simulink library "correlator_library"  (Simulink 6.2)
values from neighbouring files (symbols this model uses):
  AntBits = ceil(log2(AntNum))    [x_engine_mask.m]
  AntNum = 2    [x_engine_mask.m]
  BitGrowth = ceil(log2(AccLen))    [x_engine_mask.m]
undefined symbols (not defined in the file or in its folder): AccLen, add_latency, BitWidthIn, BitWidthOut, mult_latency
libraries: xbsIndex_r3 x745, correlator_library x7, delay_lib x5, xps_library x4
(part 1 of 6)
settings Model: LastModifiedBy=aparsons

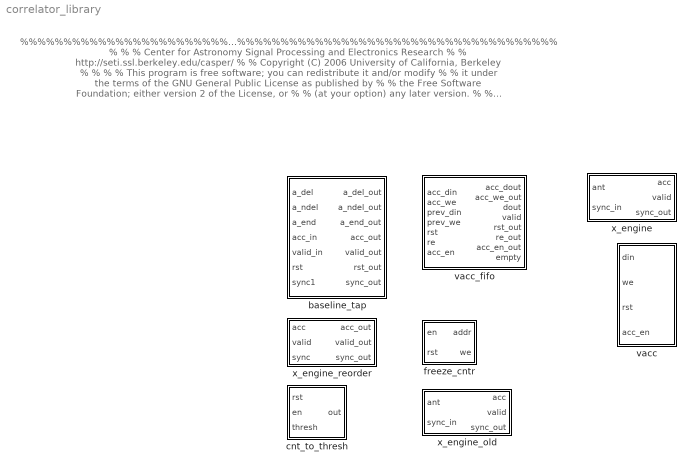
== system correlator_library ==
  note: %%%%%%%%%%%%%%%%%%%%%%%%%%%%%%%%%%%%%%%%%%%%%%%%%%%%%%%%%%%%%%%%%%%%%%%%%%%%%%%
      | %                                                                             %
      | %   Center for Astronomy Signal Processing and Electronics Research           %
      | %   http://seti.ssl.berkeley.edu/casper/                                      %
      | %   Copyright (C) 2006 University of California, Berkeley                     %
      | %                                                                             %
      | %   This program is free software; you can redistribute it and/or modify      %
      | %   it under the terms of the GNU General Public License as published by      %
      | %   the Free Software Foundation; either version 2 of the License, or         %
      | %   (at your option) any later version.                                       %
      | %                                                                             %
      | %   This program is distributed in the hope that it will be useful,           %
      | %   but WITHOUT ANY WARRANTY; without even the implied warranty of            %
      | %   MERCHANTABILITY or FITNESS FOR A PARTICULAR PURPOSE.  See the             %
      | %   GNU General Public License for more details.                              %
      | %                                                                             %
      | %   You should have received a copy of the GNU General Public License along   %
      | %   with this program; if not, write to the Free Software Foundation, Inc.,   %
      | %   51 Franklin Street, Fifth Floor, Boston, MA 02110-1301 USA.               %
      | %                                                                             %
      | %%%%%%%%%%%%%%%%%%%%%%%%%%%%%%%%%%%%%%%%%%%%%%%%%%%%%%%%%%%%%%%%%%%%%%%%%%%%%%%
  baseline_tap : Subsystem  mask(x_engine_tap){AntSep=8, use_mult_core=off, use_bram=off}
      mask prompts: AntSep "Antenna Seperation"; use_mult_core "Use Dedicated Multiplers"; use_bram "Delay in BRAM"
      mask init:
      | cursys = gcb;
      | disp(cursys);
      | multipliers = find_system(cursys, 'lookUnderMasks', 'all', 'FollowLinks','on', 'masktype', 'Xilinx Multiplier');
      | if ~strcmp(get_param(multipliers{1}, 'use_embedded'), use_mult_core),
      |     for i=1:length(multipliers),
      |         set_param(multipliers{i}, 'use_embedded', use_mult_core);
      |     end
      | end
      | if use_bram,
      |     delay_type = 'delay_bram';
      | else,
      |     delay_type = 'delay_slr';
      | end
      | if ~strcmp(get_param([cursys,'/delay'], 'BlockChoice'), delay_type),
      |     set_param([cursys,'/delay'], 'BlockChoice', delay_type)
      | end
  cnt_to_thresh : Subsystem  mask{tot_bits=0}
      mask prompts: tot_bits "Counter Bit Width"
  freeze_cntr : Subsystem  mask{CounterBits=11}
      mask prompts: CounterBits "Counter Length (2^?)"
  vacc : Subsystem  mask{vlen=8, n_bits=32, bin_pt=0, add_latency=2, arith_type=Unsigned, BitWidthIn=3, BinPtIn=0, streams=2}
      mask prompts: vlen "Vector Length"; n_bits "Output Sample Bit Width"; bin_pt "Output Binary Point"; add_latency "Add Latency"; arith_type "Arithmetic Type"; BitWidthIn "Input Bit Width"; BinPtIn "Input Binary Point"; streams "Number of Parallel Streams"
      mask init:
      | cursys = gcb;
      | disp(cursys);
      | 
      | core = [cursys,'/acc_core'];
      | if ~strcmp(get_param(core, 'arith_type'), arith_type),
      |     set_param(core, 'arith_type', arith_type);
      | end
      mask StyleString: edit,edit,edit,edit,popup(Unsigned|Signed  (2's comp)),edit,edit,edit
  vacc_fifo : Subsystem  mask(vacc_fifo){vlen=0, n_bits=0, bin_pt=0, add_latency=0, arith_type=Unsigned, BitWidthIn=0, BinPtIn=0, streams=2, stream=1}
      mask prompts: vlen "Vector Length"; n_bits "Output Sample Bit Width"; bin_pt "Output Binary Point"; add_latency "Add Latency"; arith_type "Arithmetic Type"; BitWidthIn "Input Bit Width"; BinPtIn "Input Binary Point"; streams "Number of Parallel Streams"; stream "Stream Number"
      mask init:
      | cursys = gcb;
      | disp(cursys);
      | 
      | fifo_bits = ceil(log2(max(vlen, 16)));
      | if fifo_bits >= 10,
      |     fifo_str = [num2str(2^(fifo_bits-10)), 'K'];
      | else,
      |     fifo_str = num2str(2^fifo_bits);
      | end
      | fifos = find_system(cursys, 'lookUnderMasks', 'all', 'FollowLinks','on', 'SearchDepth', 1, ...
      |     'masktype', 'Xilinx Synchronous FIFO');
      | if ~strcmp(get_param(fifos{1}, 'depth'), fifo_str),
      |     for i=1:length(fifos),
      |         set_param(fifos{i}, 'depth', fifo_str);
      |     end
      | end
      | arith_blks = {'constant', 'acc', 'reint'};
      | for i=1:length(arith_blks),
      |     name = [cursys,'/',arith_blks{i}];
      |     if ~strcmp(get_param(name, 'arith_type'), arith_type),
      |         set_param(name, 'arith_type', arith_type);
      |     end
      | end
      mask StyleString: edit,edit,edit,edit,popup(Unsigned|Signed  (2's comp)),edit,edit,edit,edit
  x_engine : Subsystem  mask{AntNum=5, BitWidthIn=8, BitWidthOut=18, AccLen=32, add_latency=1, mult_latency=1, bram_latency=1, use_mult_core=on, use_bram=off}
      mask prompts: AntNum "Number of Antennas"; BitWidthIn "Bit Width of Samples In"; BitWidthOut "Bit Width of Samples Out"; AccLen "Accumulation Length"; add_latency "Add Latency"; mult_latency "Mult Latency"; bram_latency "BRAM Latency"; use_mult_core "Use Dedicated Multipliers"; use_bram "Delay in BRAM"
      mask init:
      | x_engine_mask;
  x_engine_old : Subsystem  mask{AntNum=5, BitWidthIn=18, BitWidthOut=18, AccLen=32, add_latency=2, mult_latency=3, bram_latency=2, use_mult_core=on}
      mask prompts: AntNum "Number of Antennas"; BitWidthIn "Bit Width of Samples In"; BitWidthOut "Bit Width of Samples Out"; AccLen "Accumulation Length"; add_latency "Add Latency"; mult_latency "Mult Latency"; bram_latency "BRAM Latency"; use_mult_core "Use Dedicated Multipliers"
      mask init:
      | cursys = gcb;
      | disp(cursys);
      | set_param([cursys,'/x_engine_core'], 'use_mult_core', use_mult_core);
  x_engine_reorder : Subsystem  mask{num_ants=5, acc_len=8}
      mask prompts: num_ants "Number of Antennas"; acc_len "X Engine Accumulation Length"
      mask init:
      | num_taps = floor(num_ants/2) + 1;
      | toggle_len = num_ants * acc_len * 2;
      | 
      | addr_offset = floor(num_ants/2) * num_taps - sum(1:num_taps-1) - 1;
      | if (mod(num_ants, 2) == 0)
      |     addr_offset = addr_offset - floor(num_ants/2);
      | end
      | 
      | num_elements = nchoosek(num_ants, 2) + num_ants;
      | elements_bits = floor(log2(num_elements)) + 1;
      | %num_valids = floor(num_ants/2) + num_ants;
      | %valid_len = num_valids * acc_len;

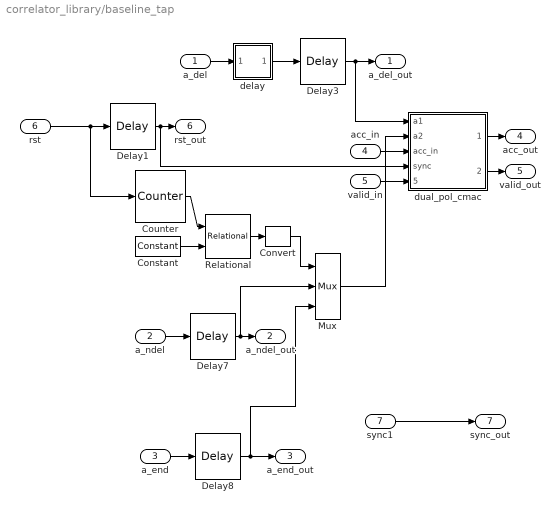
== system correlator_library/baseline_tap ==
  a_del : Inport  Port=1  LatchInput=off
  a_ndel : Inport  Port=2  LatchInput=off
  a_end : Inport  Port=3  LatchInput=off
  acc_in : Inport  Port=4  LatchInput=off
  valid_in : Inport  Port=5  LatchInput=off
  rst : Inport  Port=6  LatchInput=off
  sync1 : Inport  Port=7  LatchInput=off
  Constant : xbsIndex_r3/Constant  const=AntSep * AccLen  equ=P=C  arith_type=Unsigned  n_bits=AntBits + BitGrowth  bin_pt=0  opselect=C  inp2=PCIN>>17  opr=+  inp1=P  carry=CIN  iostate=0  explicit_period=off  period=1  dbl_ovrd=off
  Convert : xbsIndex_r3/Convert  arith_type=Unsigned  n_bits=1  bin_pt=0  quantization=Truncate  overflow=Wrap  latency=0  explicit_period=off  period=1  dbl_ovrd=off  show_param=off  inserted_by_tool=off  pipeline=off
      settings: xl_area=[0, 0, 0, 0, 0, 0, 0]
  Counter : xbsIndex_r3/Counter  cnt_type=Count Limited  n_bits=AntBits + BitGrowth  bin_pt=0  arith_type=Unsigned  start_count=0  cnt_to=AntNum * AccLen - 1  cnt_by_val=1  operation=Up  explicit_period=off  period=1  load_pin=off  rst=on  en=off  dbl_ovrd=off  show_param=off  use_rpm=on  gen_core=off
      settings: xl_area=[0, 0, 0, 0, 0, 0, 0]
  Delay1 : xbsIndex_r3/Delay  latency=1  reg_retiming=off  explicit_period=off  period=1  en=off  accept_only_valid=off  init_zero=on  dbl_ovrd=off  show_param=off
      settings: xl_area=[0, 0, 0, 0, 0, 0, 0]
  Delay3 : xbsIndex_r3/Delay  latency=1  reg_retiming=off  explicit_period=off  period=1  en=off  accept_only_valid=off  init_zero=on  dbl_ovrd=off  show_param=off
      settings: xl_area=[0, 0, 0, 0, 0, 0, 0]
  Delay7 : xbsIndex_r3/Delay  latency=1  reg_retiming=off  explicit_period=on  period=1  en=off  accept_only_valid=off  init_zero=on  dbl_ovrd=off  show_param=off
      settings: xl_area=[0, 0, 0, 0, 0, 0, 0]
  Delay8 : xbsIndex_r3/Delay  latency=1  reg_retiming=off  explicit_period=on  period=1  en=off  accept_only_valid=off  init_zero=on  dbl_ovrd=off  show_param=off
      settings: xl_area=[0, 0, 0, 0, 0, 0, 0]
  Mux : xbsIndex_r3/Mux  inputs=2  precision=Full  arith_type="Signed  (2's comp)"  n_bits=8  bin_pt=2  quantization=Truncate  overflow=Wrap  latency=0  explicit_period=off  period=1  en=off  dbl_ovrd=off  show_param=off  mux_type=off  use_rpm=off  gen_core=off
      settings: xl_area=[0, 0, 0, 0, 0, 0, 0]
  Relational : xbsIndex_r3/Relational  mode=a<b  latency=1  explicit_period=off  period=1  en=off  dbl_ovrd=off  show_param=off
      settings: xl_area=[0, 0, 0, 0, 0, 0, 0]
  delay : Subsystem  BlockChoice=delay_slr
      link override delay_bram: DelayLen=AccLen  bram_latency=bram_latency
      link override delay_bram/Constant2: equ=P=C
      link override delay_slr: DelayLen=AccLen
      settings: AttributesFormatString=%<BlockChoice>  TemplateBlock=delay_lib/delay  MemberBlocks=delay_bram,delay_slr
  dual_pol_cmac : Subsystem
  a_del_out : Outport
  a_ndel_out : Outport  Port=2
  a_end_out : Outport  Port=3
  acc_out : Outport  Port=4
  valid_out : Outport  Port=5
  rst_out : Outport  Port=6
  sync_out : Outport  Port=7
  wires:
  delay/1(Out1) -> Delay3/1
  Mux/1 -> dual_pol_cmac/2(a2)
  Counter/1 -> Relational/1
  Constant/1 -> Relational/2
  Relational/1 -> Convert/1
  Convert/1 -> Mux/1
  rst/1 -> Delay1/1, Counter/1
  a_del/1 -> delay/1(In1)
  dual_pol_cmac/1(acc_out) -> acc_out/1
  acc_in/1 -> dual_pol_cmac/3(acc_in)
  dual_pol_cmac/2(valid_out) -> valid_out/1
  valid_in/1 -> dual_pol_cmac/5(valid_in)
  a_ndel/1 -> Delay7/1
  a_end/1 -> Delay8/1
  Delay3/1 -> a_del_out/1, dual_pol_cmac/1(a1)
  Delay7/1 -> a_ndel_out/1, Mux/2
  Delay8/1 -> a_end_out/1, Mux/3
  Delay1/1 -> rst_out/1, dual_pol_cmac/4(sync)
  sync1/1 -> sync_out/1

== system correlator_library/cnt_to_thresh ==
  rst : Inport  Port=1  LatchInput=off
  en : Inport  Port=2  LatchInput=off
  thresh : Inport  Port=3  LatchInput=off
  Inverter : xbsIndex_r3/Inverter  latency=0  explicit_period=off  period=1  en=off  dbl_ovrd=off  show_param=off
      settings: xl_area=[0, 0, 0, 0, 0, 0, 0]
  Logical : xbsIndex_r3/Logical  logical_function=AND  inputs=3  precision=Full  arith_type=Unsigned  n_bits=8  bin_pt=2  align_bp=on  latency=0  explicit_period=off  period=1  en=off  dbl_ovrd=off  show_param=off
      settings: xl_area=[0, 0, 0, 0, 0, 0, 0]
  Logical1 : xbsIndex_r3/Logical  logical_function=OR  inputs=2  precision=Full  arith_type=Unsigned  n_bits=8  bin_pt=2  align_bp=on  latency=0  explicit_period=off  period=1  en=off  dbl_ovrd=off  show_param=off
      settings: xl_area=[0, 0, 0, 0, 0, 0, 0]
  Relational1 : xbsIndex_r3/Relational  mode=a>=b  latency=2  explicit_period=on  period=1  en=on  dbl_ovrd=off  show_param=off
      settings: xl_area=[0, 0, 0, 0, 0, 0, 0]
  accumulator_adder1 : xbsIndex_r3/AddSub  mode=Subtraction  precision=User Defined  arith_type=Unsigned  n_bits=tot_bits  bin_pt=0  quantization=Truncate  overflow=Wrap  latency=add_latency  explicit_period=on  period=1  use_carryin=off  use_carryout=off  en=off  dbl_ovrd=off  show_param=off  use_core=on  pipeline=off  use_rpm=on  gen_core=off
      settings: xl_area=[0, 0, 0, 0, 0, 0, 0]
  accumulator_address_delay : xbsIndex_r3/Delay  latency=1  reg_retiming=off  explicit_period=off  period=1  en=on  accept_only_valid=off  init_zero=on  dbl_ovrd=off  show_param=off
      settings: xl_area=[0, 0, 0, 0, 0, 0, 0]
  const_accumulator_data_reset1 : xbsIndex_r3/Constant  const=2 + 1  equ=P=C  arith_type=Unsigned  n_bits=n_bits  bin_pt=0  opselect=C  inp2=PCIN>>17  opr=+  inp1=P  carry=CIN  iostate=0  explicit_period=on  period=1  dbl_ovrd=off
  int_cnt : xbsIndex_r3/Counter  cnt_type=Free Running  n_bits=tot_bits  bin_pt=0  arith_type=Unsigned  start_count=0  cnt_to=Inf  cnt_by_val=1  operation=Up  explicit_period=off  period=1  load_pin=off  rst=on  en=on  dbl_ovrd=off  show_param=off  use_rpm=on  gen_core=off
      settings: xl_area=[0, 0, 0, 0, 0, 0, 0]
  out : Outport
  wires:
  Inverter/1 -> Logical/2
  accumulator_address_delay/1 -> Inverter/1
  Logical1/1 -> int_cnt/1
  int_cnt/1 -> Relational1/1, out/1
  accumulator_adder1/1 -> Relational1/2
  const_accumulator_data_reset1/1 -> accumulator_adder1/2
  rst/1 -> Logical1/2
  en/1 -> accumulator_address_delay/2, Logical/3, int_cnt/2, Relational1/3
  thresh/1 -> accumulator_adder1/1
  Logical/1 -> Logical1/1
  Relational1/1 -> accumulator_address_delay/1, Logical/1

== system correlator_library/freeze_cntr ==
  en : Inport  Port=1  LatchInput=off
  rst : Inport  Port=2  LatchInput=off
  Constant5 : xbsIndex_r3/Constant  const=2^CounterBits - 1  equ=P=C  arith_type=Unsigned  n_bits=CounterBits  bin_pt=0  opselect=C  inp2=PCIN>>17  opr=+  inp1=P  carry=CIN  iostate=0  explicit_period=off  period=1  dbl_ovrd=off
  Counter3 : xbsIndex_r3/Counter  cnt_type=Free Running  n_bits=CounterBits  bin_pt=0  arith_type=Unsigned  start_count=0  cnt_to=1023  cnt_by_val=1  operation=Up  explicit_period=on  period=1  load_pin=off  rst=on  en=on  dbl_ovrd=off  show_param=off  use_rpm=on  gen_core=off
      settings: xl_area=[0, 0, 0, 0, 0, 0, 0]
  Inverter : xbsIndex_r3/Inverter  latency=0  explicit_period=off  period=1  en=off  dbl_ovrd=off  show_param=off
      settings: xl_area=[0, 0, 0, 0, 0, 0, 0]
  Logical1 : xbsIndex_r3/Logical  logical_function=AND  inputs=2  precision=Full  arith_type=Unsigned  n_bits=8  bin_pt=2  align_bp=on  latency=0  explicit_period=off  period=1  en=off  dbl_ovrd=off  show_param=off
      settings: xl_area=[0, 0, 0, 0, 0, 0, 0]
  Logical5 : xbsIndex_r3/Logical  logical_function=AND  inputs=2  precision=Full  arith_type=Unsigned  n_bits=8  bin_pt=2  align_bp=on  latency=0  explicit_period=off  period=1  en=off  dbl_ovrd=off  show_param=off
      settings: xl_area=[0, 0, 0, 0, 0, 0, 0]
  Relational5 : xbsIndex_r3/Relational  mode=a!=b  latency=0  explicit_period=off  period=1  en=off  dbl_ovrd=off  show_param=off
      settings: xl_area=[0, 0, 0, 0, 0, 0, 0]
  addr : Outport
  we : Outport  Port=2
  wires:
  Logical1/1 -> we/1
  Inverter/1 -> Logical1/1
  Counter3/1 -> addr/1, Relational5/1
  Constant5/1 -> Relational5/2
  Relational5/1 -> Logical5/2
  en/1 -> Logical5/1
  Logical5/1 -> Logical1/2, Counter3/2
  rst/1 -> Inverter/1, Counter3/1

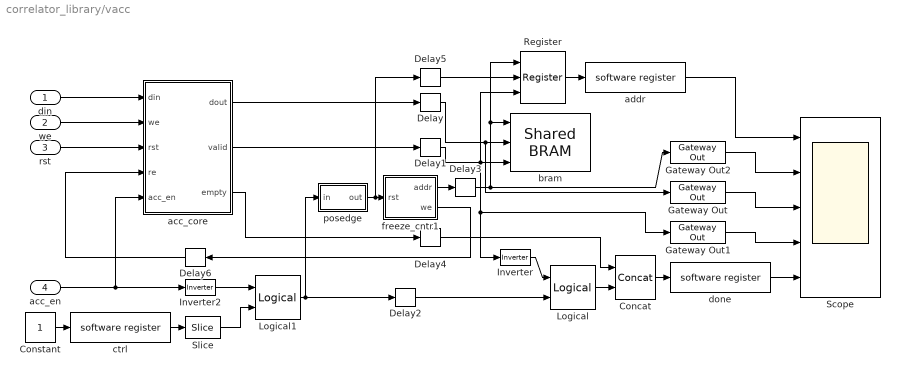
== system correlator_library/vacc ==
  din : Inport  Port=1  LatchInput=off
  we : Inport  Port=2  LatchInput=off
  rst : Inport  Port=3  LatchInput=off
  acc_en : Inport  Port=4  LatchInput=off
  Concat : xbsIndex_r3/Concat  num_inputs=2  explicit_period=off  period=1  dbl_ovrd=off
  Constant : Constant
  Delay : xbsIndex_r3/Delay  latency=1  reg_retiming=off  explicit_period=off  period=1  en=off  accept_only_valid=off  init_zero=on  dbl_ovrd=off  show_param=off
      settings: xl_area=[0, 0, 0, 0, 0, 0, 0]
  Delay1 : xbsIndex_r3/Delay  latency=1  reg_retiming=off  explicit_period=off  period=1  en=off  accept_only_valid=off  init_zero=on  dbl_ovrd=off  show_param=off
      settings: xl_area=[0, 0, 0, 0, 0, 0, 0]
  Delay2 : xbsIndex_r3/Delay  latency=6  reg_retiming=off  explicit_period=off  period=1  en=off  accept_only_valid=off  init_zero=on  dbl_ovrd=off  show_param=off
      settings: xl_area=[0, 0, 0, 0, 0, 0, 0]
  Delay3 : xbsIndex_r3/Delay  latency=4  reg_retiming=off  explicit_period=off  period=1  en=off  accept_only_valid=off  init_zero=on  dbl_ovrd=off  show_param=off
      settings: xl_area=[0, 0, 0, 0, 0, 0, 0]
  Delay4 : xbsIndex_r3/Delay  latency=2  reg_retiming=off  explicit_period=on  period=1  en=off  accept_only_valid=off  init_zero=on  dbl_ovrd=off  show_param=off
      settings: xl_area=[0, 0, 0, 0, 0, 0, 0]
  Delay5 : xbsIndex_r3/Delay  latency=3  reg_retiming=off  explicit_period=off  period=1  en=off  accept_only_valid=off  init_zero=on  dbl_ovrd=off  show_param=off
      settings: xl_area=[0, 0, 0, 0, 0, 0, 0]
  Delay6 : xbsIndex_r3/Delay  Orientation=left  latency=3  reg_retiming=off  explicit_period=off  period=1  en=off  accept_only_valid=off  init_zero=on  dbl_ovrd=off  show_param=off
      settings: xl_area=[0, 0, 0, 0, 0, 0, 0]
  Gateway Out : xbsIndex_r3/Gateway Out  output_type=Double  nbits=8  bin_pt=6  arith_type=Boolean  quantization=Truncate  overflow=Wrap  hdl_port=off  timing_constraint=None  locs_specified=off  LOCs={}  needs_fixed_name=off  show_param=off
      settings: xl_area=[0, 0, 0, 0, 0, 0, 0]
  Gateway Out1 : xbsIndex_r3/Gateway Out  output_type=Double  nbits=8  bin_pt=6  arith_type=Boolean  quantization=Truncate  overflow=Wrap  hdl_port=off  timing_constraint=None  locs_specified=off  LOCs={}  needs_fixed_name=off  show_param=off
      settings: xl_area=[0, 0, 0, 0, 0, 0, 0]
  Gateway Out2 : xbsIndex_r3/Gateway Out  output_type=Double  nbits=8  bin_pt=6  arith_type=Boolean  quantization=Truncate  overflow=Wrap  hdl_port=off  timing_constraint=None  locs_specified=off  LOCs={}  needs_fixed_name=off  show_param=off
      settings: xl_area=[0, 0, 0, 0, 0, 0, 0]
  Inverter : xbsIndex_r3/Inverter  latency=0  explicit_period=off  period=1  en=off  dbl_ovrd=off  show_param=off
      settings: xl_area=[0, 0, 0, 0, 0, 0, 0]
  Inverter2 : xbsIndex_r3/Inverter  latency=0  explicit_period=off  period=1  en=off  dbl_ovrd=off  show_param=off
      settings: xl_area=[0, 0, 0, 0, 0, 0, 0]
  Logical : xbsIndex_r3/Logical  logical_function=AND  inputs=2  precision=Full  arith_type=Unsigned  n_bits=8  bin_pt=2  align_bp=on  latency=0  explicit_period=off  period=1  en=off  dbl_ovrd=off  show_param=off
      settings: xl_area=[0, 0, 0, 0, 0, 0, 0]
  Logical1 : xbsIndex_r3/Logical  logical_function=AND  inputs=2  precision=Full  arith_type=Unsigned  n_bits=8  bin_pt=2  align_bp=on  latency=1  explicit_period=off  period=1  en=off  dbl_ovrd=off  show_param=off
      settings: xl_area=[0, 0, 0, 0, 0, 0, 0]
  Register : xbsIndex_r3/Register  init=0  reg_only_valid=off  explicit_period=off  period=1  rst=on  en=on  out_en=off  dbl_ovrd=off  show_param=off
      settings: xl_area=[0, 0, 0, 0, 0, 0, 0]
  Scope : Scope  NumInputPorts=5
      settings: YMin=0~-2250~0~-5~-5  YMax=2250~2250~1~5~5
  Slice : xbsIndex_r3/Slice  mode=Lower Bit Location + Width  nbits=1  bit1=0  base1=MSB of Input  bit0=0  base0=LSB of Input  boolean_output=on  explicit_period=off  period=1  dbl_ovrd=off
  acc_core : Subsystem  mask{vlen=vlen, n_bits=n_bits, bin_pt=bin_pt, add_latency=add_latency, arith_type=Unsigned, BitWidthIn=BitWidthIn, BinPtIn=BinPtIn, streams=streams}
      mask prompts: vlen "Vector Length"; n_bits "Output Sample Bit Width"; bin_pt "Output Binary Point"; add_latency "Add Latency"; arith_type "Arithmetic Type"; BitWidthIn "Input Bit Width"; BinPtIn "Input Binary Point"; streams "Number of Parallel Streams"
      mask init:
      | acc_core_mask;
      mask StyleString: edit,edit,edit,edit,popup(Unsigned|Signed  (2's comp)),edit,edit,edit
  addr : xps_library/software register  Tag=xps:sw_reg  io_dir=To Processor  arith_type=Unsigned  bitwidth=32  bin_pt=0  sample_period=1  gw_name=correlator_library_vacc_addr_user_data_in
  bram : xps_library/Shared BRAM  Tag=xps:bram  arith_type="Signed  (2's comp)"  addr_width=11  data_width=32  data_bin_pt=bin_pt  init_vals=0  sample_rate=1
  ctrl : xps_library/software register  Tag=xps:sw_reg  io_dir=From Processor  arith_type=Unsigned  bitwidth=32  bin_pt=0  sample_period=1  gw_name=correlator_library_vacc_ctrl_user_data_out
  done : xps_library/software register  Tag=xps:sw_reg  io_dir=To Processor  arith_type=Unsigned  bitwidth=32  bin_pt=0  sample_period=1  gw_name=correlator_library_vacc_done_user_data_in
  freeze_cntr1 : Subsystem  mask{CounterBits=11}
      mask prompts: CounterBits "Counter Length (2^?)"
  posedge : Subsystem
  wires:
  Gateway Out2/1 -> Scope/2
  addr/1 -> Scope/1
  Gateway Out/1 -> Scope/3
  Gateway Out1/1 -> Scope/4
  done/1 -> Scope/5
  posedge/1(out) -> freeze_cntr1/1(rst), Delay5/1
  Logical1/1 -> posedge/1(in), Delay2/1
  Inverter2/1 -> Logical1/1
  Slice/1 -> Logical1/2
  ctrl/1 -> Slice/1
  acc_en/1 -> Inverter2/1, acc_core/5(acc_en)
  Inverter/1 -> Logical/1
  acc_core/1(dout) -> Delay/1
  freeze_cntr1/2(we) -> Delay6/1
  freeze_cntr1/1(addr) -> Delay3/1
  acc_core/2(valid) -> Delay1/1
  rst/1 -> acc_core/3(rst)
  we/1 -> acc_core/2(we)
  din/1 -> acc_core/1(din)
  Delay/1 -> bram/2, Gateway Out/1
  Constant/1 -> ctrl/1
  Delay1/1 -> Gateway Out1/1, Inverter/1, bram/3, Register/3
  Delay2/1 -> Logical/2
  Delay3/1 -> Gateway Out2/1, bram/1, Register/1
  Register/1 -> addr/1
  acc_core/3(empty) -> Delay4/1
  Logical/1 -> Concat/2
  Concat/1 -> done/1
  Delay4/1 -> Concat/1
  Delay6/1 -> acc_core/4(re)
  Delay5/1 -> Register/2

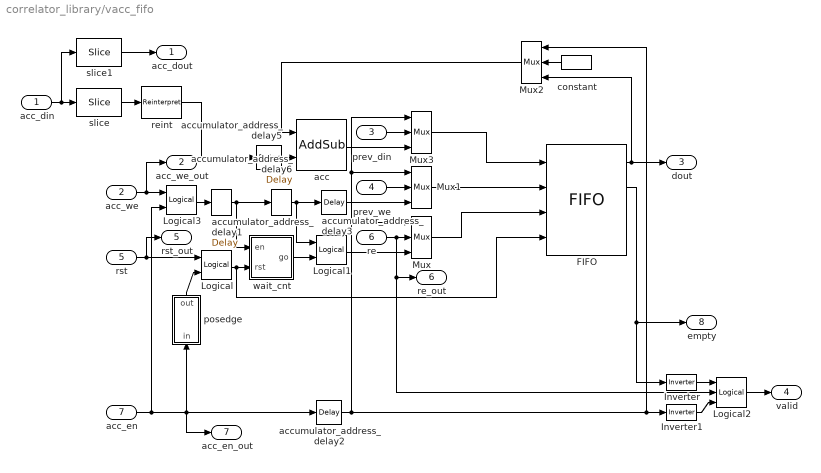
== system correlator_library/vacc_fifo ==
  acc_din : Inport  Port=1  LatchInput=off
  acc_we : Inport  Port=2  LatchInput=off
  prev_din : Inport  Port=3  LatchInput=off
  prev_we : Inport  Port=4  LatchInput=off
  rst : Inport  Port=5  LatchInput=off
  re : Inport  Port=6  LatchInput=off
  acc_en : Inport  Port=7  LatchInput=off
  FIFO : xbsIndex_r3/FIFO  depth=16  percent_nbits=1  store_only_valid=on  init_zero=on  explicit_period=on  period=1  rst=on  en=off  use_almost_empty=off  almost_empty_offset=6  use_almost_full=off  almost_full_offset=6  dbl_ovrd=off  show_param=off  mem_type=Block RAM  gen_core=off
      settings: xl_area=[0, 0, 0, 0, 0, 0, 0]
  Inverter : xbsIndex_r3/Inverter  latency=1  explicit_period=off  period=1  en=off  dbl_ovrd=off  show_param=off
      settings: xl_area=[0, 0, 0, 0, 0, 0, 0]
  Inverter1 : xbsIndex_r3/Inverter  latency=0  explicit_period=off  period=1  en=off  dbl_ovrd=off  show_param=off
      settings: xl_area=[0, 0, 0, 0, 0, 0, 0]
  Logical : xbsIndex_r3/Logical  logical_function=OR  inputs=2  precision=Full  arith_type=Unsigned  n_bits=8  bin_pt=2  align_bp=on  latency=0  explicit_period=off  period=1  en=off  dbl_ovrd=off  show_param=off
      settings: xl_area=[0, 0, 0, 0, 0, 0, 0]
  Logical1 : xbsIndex_r3/Logical  logical_function=AND  inputs=2  precision=Full  arith_type=Unsigned  n_bits=8  bin_pt=2  align_bp=on  latency=0  explicit_period=off  period=1  en=off  dbl_ovrd=off  show_param=off
      settings: xl_area=[0, 0, 0, 0, 0, 0, 0]
  Logical2 : xbsIndex_r3/Logical  logical_function=AND  inputs=3  precision=Full  arith_type=Unsigned  n_bits=8  bin_pt=2  align_bp=on  latency=0  explicit_period=off  period=1  en=off  dbl_ovrd=off  show_param=off
      settings: xl_area=[0, 0, 0, 0, 0, 0, 0]
  Logical3 : xbsIndex_r3/Logical  logical_function=AND  inputs=2  precision=Full  arith_type=Unsigned  n_bits=8  bin_pt=2  align_bp=on  latency=0  explicit_period=off  period=1  en=off  dbl_ovrd=off  show_param=off
      settings: xl_area=[0, 0, 0, 0, 0, 0, 0]
  Mux : xbsIndex_r3/Mux  inputs=2  precision=Full  arith_type="Signed  (2's comp)"  n_bits=8  bin_pt=2  quantization=Truncate  overflow=Wrap  latency=0  explicit_period=off  period=1  en=off  dbl_ovrd=off  show_param=off  mux_type=off  use_rpm=off  gen_core=off
      settings: xl_area=[0, 0, 0, 0, 0, 0, 0]
  Mux1 : xbsIndex_r3/Mux  inputs=2  precision=Full  arith_type="Signed  (2's comp)"  n_bits=8  bin_pt=2  quantization=Truncate  overflow=Wrap  latency=0  explicit_period=off  period=1  en=off  dbl_ovrd=off  show_param=off  mux_type=off  use_rpm=off  gen_core=off
      settings: xl_area=[0, 0, 0, 0, 0, 0, 0]
  Mux2 : xbsIndex_r3/Mux  Orientation=left  inputs=2  precision=Full  arith_type="Signed  (2's comp)"  n_bits=8  bin_pt=2  quantization=Truncate  overflow=Wrap  latency=0  explicit_period=off  period=1  en=off  dbl_ovrd=off  show_param=off  mux_type=off  use_rpm=off  gen_core=off
      settings: xl_area=[0, 0, 0, 0, 0, 0, 0]
  Mux3 : xbsIndex_r3/Mux  inputs=2  precision=Full  arith_type="Signed  (2's comp)"  n_bits=8  bin_pt=2  quantization=Truncate  overflow=Wrap  latency=0  explicit_period=off  period=1  en=off  dbl_ovrd=off  show_param=off  mux_type=off  use_rpm=off  gen_core=off
      settings: xl_area=[0, 0, 0, 0, 0, 0, 0]
  acc : xbsIndex_r3/AddSub  mode=Addition  precision=User Defined  arith_type=Unsigned  n_bits=n_bits  bin_pt=bin_pt  quantization="Round  (unbiased: +/- Inf)"  overflow=Wrap  latency=add_latency  explicit_period=on  period=1  use_carryin=off  use_carryout=off  en=off  dbl_ovrd=off  show_param=off  use_core=on  pipeline=off  use_rpm=on  gen_core=off
      settings: xl_area=[0, 0, 0, 0, 0, 0, 0]
  accumulator_address_delay1 : xbsIndex_r3/Delay  latency=1  reg_retiming=off  explicit_period=off  period=1  en=off  accept_only_valid=off  init_zero=on  dbl_ovrd=off  show_param=off
      settings: xl_area=[0, 0, 0, 0, 0, 0, 0]
  accumulator_address_delay2 : xbsIndex_r3/Delay  latency=add_latency + 2  reg_retiming=off  explicit_period=off  period=1  en=off  accept_only_valid=off  init_zero=on  dbl_ovrd=off  show_param=off
      settings: xl_area=[0, 0, 0, 0, 0, 0, 0]
  accumulator_address_delay3 : xbsIndex_r3/Delay  latency=add_latency  reg_retiming=off  explicit_period=off  period=1  en=off  accept_only_valid=off  init_zero=on  dbl_ovrd=off  show_param=off
      settings: xl_area=[0, 0, 0, 0, 0, 0, 0]
  accumulator_address_delay5 : xbsIndex_r3/Delay  latency=2  reg_retiming=off  explicit_period=off  period=1  en=off  accept_only_valid=off  init_zero=on  dbl_ovrd=off  show_param=off
      settings: xl_area=[0, 0, 0, 0, 0, 0, 0]
  accumulator_address_delay6 : xbsIndex_r3/Delay  latency=1  reg_retiming=off  explicit_period=off  period=1  en=off  accept_only_valid=off  init_zero=on  dbl_ovrd=off  show_param=off
      settings: xl_area=[0, 0, 0, 0, 0, 0, 0]
  constant : xbsIndex_r3/Constant  Orientation=left  const=0  equ=P=C  arith_type=Unsigned  n_bits=n_bits  bin_pt=bin_pt  opselect=C  inp2=PCIN>>17  opr=+  inp1=P  carry=CIN  iostate=0  explicit_period=on  period=1  dbl_ovrd=off
  posedge : Subsystem  Orientation=up
  reint : xbsIndex_r3/Reinterpret  force_arith_type=on  arith_type=Unsigned  force_bin_pt=on  bin_pt=BinPtIn  force_valid=on
  slice : xbsIndex_r3/Slice  mode=Lower Bit Location + Width  nbits=BitWidthIn  bit1=0  base1=MSB of Input  bit0=0  base0=LSB of Input  boolean_output=off  explicit_period=off  period=1  dbl_ovrd=off
  slice1 : xbsIndex_r3/Slice  mode=Two Bit Locations  nbits=n_bits  bit1=0  base1=MSB of Input  bit0=min(BitWidthIn, (streams-stream)*BitWidthIn)  base0=LSB of Input  boolean_output=off  explicit_period=off  period=1  dbl_ovrd=off
  wait_cnt : Subsystem
  acc_dout : Outport
  acc_we_out : Outport  Port=2
  dout : Outport  Port=3
  valid : Outport  Port=4
  rst_out : Outport  Port=5
  re_out : Outport  Port=6
  acc_en_out : Outport  Port=7
  empty : Outport  Port=8
  wires:
  prev_we/1 -> Mux1/2
  Logical2/1 -> valid/1
  Inverter/1 -> Logical2/1
  re/1 -> Mux/2, Logical2/2, re_out/1
  prev_din/1 -> Mux3/2
  Mux1/1 -> FIFO/2
  acc/1 -> Mux3/3
  accumulator_address_delay3/1 -> Mux1/3
  Mux/1 -> FIFO/3
  acc_en/1 -> posedge/1(in), accumulator_address_delay2/1, acc_en_out/1, Logical3/2
  Logical/1 -> wait_cnt/2(rst), FIFO/4
  rst/1 -> Logical/1, rst_out/1
  posedge/1(out) -> Logical/2
  Logical1/1 -> Mux/3
  wait_cnt/1(go) -> Logical1/2
  Logical3/1 -> accumulator_address_delay1/1
  Mux2/1 -> acc/1
  constant/1 -> Mux2/2
  acc_we/1 -> Logical3/1, acc_we_out/1
  accumulator_address_delay5/1 -> acc/2
  accumulator_address_delay1/1 -> wait_cnt/1(en), accumulator_address_delay6/1
  accumulator_address_delay6/1 -> accumulator_address_delay3/1, Logical1/1
  accumulator_address_delay2/1 -> Mux/1, Mux1/1, Mux3/1, Mux2/1, Inverter1/1
  Inverter1/1 -> Logical2/3
  Mux3/1 -> FIFO/1
  FIFO/2 -> Inverter/1, empty/1
  FIFO/1 -> Mux2/3, dout/1
  slice/1 -> reint/1
  acc_din/1 -> slice/1, slice1/1
  reint/1 -> accumulator_address_delay5/1
  slice1/1 -> acc_dout/1

== system correlator_library/x_engine ==
  ant : Inport  Port=1  LatchInput=off
  sync_in : Inport  Port=2  LatchInput=off
  Constant : xbsIndex_r3/Constant  const=0  equ=P=C  arith_type=Unsigned  n_bits=8 * BitWidthOut  bin_pt=0  opselect=C  inp2=PCIN>>17  opr=+  inp1=P  carry=CIN  iostate=0  explicit_period=on  period=1  dbl_ovrd=off
  Constant1 : xbsIndex_r3/Constant  const=0  equ=P=C  arith_type=Boolean  n_bits=1  bin_pt=0  opselect=C  inp2=PCIN>>17  opr=+  inp1=P  carry=CIN  iostate=0  explicit_period=on  period=1  dbl_ovrd=off
  Term1 : Terminator
  Term2 : Terminator
  Term3 : Terminator
  auto_tap : Subsystem  mask(x_engine_tap){use_mult_core=on, use_bram=off}
      mask prompts: use_mult_core "Use Dedicated Multipliers"; use_bram "Delay in BRAM"
      mask init:
      | cursys = gcb;
      | disp(cursys);
      | multipliers = find_system(cursys, 'lookUnderMasks', 'all', 'FollowLinks','on', 'masktype', 'Xilinx Multiplier');
      | if ~strcmp(get_param(multipliers{1}, 'use_embedded'), use_mult_core),
      |     for i=1:length(multipliers),
      |         set_param(multipliers{i}, 'use_embedded', use_mult_core);
      |     end
      | end
      | 
      | %if use_mult_core, mc = 'on';
      | %else, mc = 'off';
      | %end
      | %for i=1:length(multipliers),
      | %    m = multipliers{i};
      | %    if ~strcmp(get_param(m, 'use_embedded'), mc),
      | %        set_param(m, 'use_embedded', mc);
      | %    end
      | %end
  baseline_tap1 : correlator_library/baseline_tap  AntSep=1  use_mult_core=on  use_bram=off
  baseline_tap2 : correlator_library/baseline_tap  AntSep=2  use_mult_core=on  use_bram=off
  acc : Outport
  valid : Outport  Port=2
  sync_out : Outport  Port=3
  wires:
  ant/1 -> auto_tap/1(a_del), auto_tap/2(a_ndel)
  Constant/1 -> auto_tap/4(acc_in)
  Constant1/1 -> auto_tap/5(valid_in)
  sync_in/1 -> auto_tap/6(sync_in)
  auto_tap/1(a_del_out) -> baseline_tap1/1
  auto_tap/2(a_ndel_out) -> baseline_tap1/2
  auto_tap/3(a_end_out) -> baseline_tap1/3
  auto_tap/4(acc_out) -> baseline_tap1/4
  auto_tap/5(valid_out) -> baseline_tap1/5
  auto_tap/6(rst_out) -> baseline_tap1/6
  auto_tap/7(sync_out) -> baseline_tap1/7
  baseline_tap1/1 -> baseline_tap2/1
  baseline_tap1/2 -> baseline_tap2/2
  baseline_tap1/3 -> baseline_tap2/3
  baseline_tap1/4 -> baseline_tap2/4
  baseline_tap1/5 -> baseline_tap2/5
  baseline_tap1/6 -> baseline_tap2/6
  baseline_tap1/7 -> baseline_tap2/7
  baseline_tap2/1 -> auto_tap/3(a_loop)
  baseline_tap2/2 -> Term1/1
  baseline_tap2/3 -> Term2/1
  baseline_tap2/4 -> acc/1
  baseline_tap2/5 -> valid/1
  baseline_tap2/6 -> Term3/1
  baseline_tap2/7 -> sync_out/1

== system correlator_library/x_engine_old ==
  ant : Inport  Port=1  LatchInput=off
  sync_in : Inport  Port=2  LatchInput=off
  x_engine_core : Subsystem  mask{AntNum=AntNum, BitWidthIn=BitWidthIn, BitWidthOut=BitWidthOut, AccLen=AccLen, add_latency=add_latency, mult_latency=mult_latency, bram_latency=bram_latency, use_mult_core=on}
      mask prompts: AntNum "Number of Antennas"; BitWidthIn "Bit Width of Samples In"; BitWidthOut "Bit Width of Samples Out"; AccLen "Accumulation Length"; add_latency "Add Latency"; mult_latency "Mult Latency"; bram_latency "BRAM Latency"; use_mult_core "Use Dedicated Multipliers"
      mask init:
      | x_engine_mask;
  acc : Outport
  valid : Outport  Port=2
  sync_out : Outport  Port=3
  wires:
  x_engine_core/3(sync_out) -> sync_out/1
  x_engine_core/1(acc) -> acc/1
  ant/1 -> x_engine_core/1(ant)
  x_engine_core/2(valid) -> valid/1
  sync_in/1 -> x_engine_core/2(sync_in)

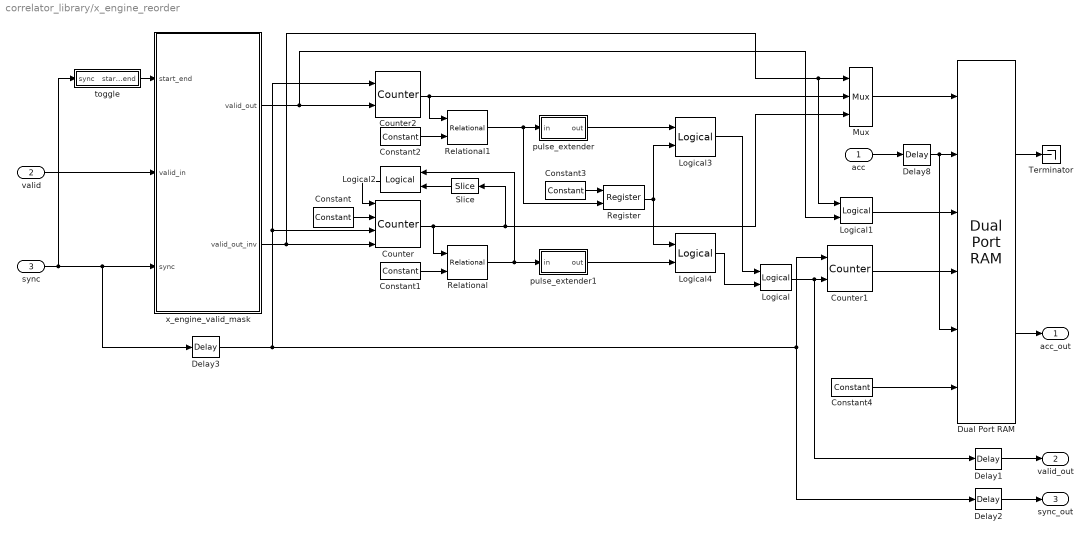
== system correlator_library/x_engine_reorder ==
  acc : Inport  Port=1  LatchInput=off
  valid : Inport  Port=2  LatchInput=off
  sync : Inport  Port=3  LatchInput=off
  Constant : xbsIndex_r3/Constant  const=num_elements  equ=P=C  arith_type=Unsigned  n_bits=elements_bits + 1  bin_pt=0  opselect=C  inp2=PCIN>>17  opr=+  inp1=P  carry=CIN  iostate=0  explicit_period=on  period=1  dbl_ovrd=off
  Constant1 : xbsIndex_r3/Constant  const=num_elements * 2 - 2  equ=P=C  arith_type=Unsigned  n_bits=elements_bits + 1  bin_pt=0  opselect=C  inp2=PCIN>>17  opr=+  inp1=P  carry=CIN  iostate=0  explicit_period=on  period=1  dbl_ovrd=off
  Constant2 : xbsIndex_r3/Constant  const=num_elements - 1  equ=P=C  arith_type=Unsigned  n_bits=elements_bits + 1  bin_pt=0  opselect=C  inp2=PCIN>>17  opr=+  inp1=P  carry=CIN  iostate=0  explicit_period=on  period=1  dbl_ovrd=off
  Constant3 : xbsIndex_r3/Constant  const=1  equ=P=C  arith_type=Boolean  n_bits=elements_bits + 1  bin_pt=0  opselect=C  inp2=PCIN>>17  opr=+  inp1=P  carry=CIN  iostate=0  explicit_period=on  period=1  dbl_ovrd=off
  Constant4 : xbsIndex_r3/Constant  const=0  equ=P=C  arith_type=Boolean  n_bits=elements_bits + 1  bin_pt=0  opselect=C  inp2=PCIN>>17  opr=+  inp1=P  carry=CIN  iostate=0  explicit_period=on  period=1  dbl_ovrd=off
  Counter : xbsIndex_r3/Counter  cnt_type=Free Running  n_bits=elements_bits + 1  bin_pt=0  arith_type=Unsigned  start_count=num_elements * 2 - 1 - addr_offset  cnt_to=71  cnt_by_val=1  operation=Up  explicit_period=off  period=1  load_pin=on  rst=on  en=on  dbl_ovrd=off  show_param=off  use_rpm=on  gen_core=off
      settings: xl_area=[0, 0, 0, 0, 0, 0, 0]
  Counter1 : xbsIndex_r3/Counter  cnt_type=Count Limited  n_bits=elements_bits + 1  bin_pt=0  arith_type=Unsigned  start_count=0  cnt_to=2 * num_elements - 1  cnt_by_val=1  operation=Up  explicit_period=off  period=1  load_pin=off  rst=on  en=on  dbl_ovrd=off  show_param=off  use_rpm=on  gen_core=off
      settings: xl_area=[0, 0, 0, 0, 0, 0, 0]
  Counter2 : xbsIndex_r3/Counter  cnt_type=Count Limited  n_bits=elements_bits + 1  bin_pt=0  arith_type=Unsigned  start_count=0  cnt_to=num_elements - 1  cnt_by_val=1  operation=Up  explicit_period=off  period=1  load_pin=off  rst=on  en=on  dbl_ovrd=off  show_param=off  use_rpm=on  gen_core=off
      settings: xl_area=[0, 0, 0, 0, 0, 0, 0]
  Delay1 : xbsIndex_r3/Delay  latency=1  reg_retiming=off  explicit_period=off  period=1  en=off  accept_only_valid=off  init_zero=on  dbl_ovrd=off  show_param=off
      settings: xl_area=[0, 0, 0, 0, 0, 0, 0]
  Delay2 : xbsIndex_r3/Delay  latency=1  reg_retiming=off  explicit_period=off  period=1  en=off  accept_only_valid=off  init_zero=on  dbl_ovrd=off  show_param=off
      settings: xl_area=[0, 0, 0, 0, 0, 0, 0]
  Delay3 : xbsIndex_r3/Delay  latency=2  reg_retiming=off  explicit_period=off  period=1  en=off  accept_only_valid=off  init_zero=on  dbl_ovrd=off  show_param=off
      settings: xl_area=[0, 0, 0, 0, 0, 0, 0]
  Delay8 : xbsIndex_r3/Delay  latency=2  reg_retiming=off  explicit_period=off  period=1  en=off  accept_only_valid=off  init_zero=on  dbl_ovrd=off  show_param=off
      settings: xl_area=[0, 0, 0, 0, 0, 0, 0]
  Dual Port RAM : xbsIndex_r3/Dual Port RAM  depth=num_elements * 2  initVector=sin(pi*(0:num_elements * 2 - 1)/num_elements * 2)  write_mode_A=Read After Write  write_mode_B=No Read On Write  latency=1  mem_collision=off  init_zero=on  explicit_period=off  period=1  dbl_ovrd=off  rst_a=off  init_a=0  rst_b=off  init_b=0  show_param=off  distributed_mem=off  use_rpm=off  gen_core=off
      settings: xl_area=[0, 0, 0, 0, 0, 0, 0]
  Logical : xbsIndex_r3/Logical  logical_function=OR  inputs=2  precision=Full  arith_type=Unsigned  n_bits=8  bin_pt=2  align_bp=on  latency=0  explicit_period=off  period=1  en=off  dbl_ovrd=off  show_param=off
      settings: xl_area=[0, 0, 0, 0, 0, 0, 0]
  Logical1 : xbsIndex_r3/Logical  logical_function=OR  inputs=2  precision=Full  arith_type=Unsigned  n_bits=8  bin_pt=2  align_bp=on  latency=0  explicit_period=off  period=1  en=off  dbl_ovrd=off  show_param=off
      settings: xl_area=[0, 0, 0, 0, 0, 0, 0]
  Logical2 : xbsIndex_r3/Logical  Orientation=left  logical_function=AND  inputs=2  precision=Full  arith_type=Unsigned  n_bits=8  bin_pt=2  align_bp=on  latency=0  explicit_period=on  period=1  en=off  dbl_ovrd=off  show_param=off
      settings: xl_area=[0, 0, 0, 0, 0, 0, 0]
  Logical3 : xbsIndex_r3/Logical  logical_function=AND  inputs=2  precision=Full  arith_type=Unsigned  n_bits=8  bin_pt=2  align_bp=on  latency=0  explicit_period=off  period=1  en=off  dbl_ovrd=off  show_param=off
      settings: xl_area=[0, 0, 0, 0, 0, 0, 0]
  Logical4 : xbsIndex_r3/Logical  logical_function=AND  inputs=2  precision=Full  arith_type=Unsigned  n_bits=8  bin_pt=2  align_bp=on  latency=0  explicit_period=off  period=1  en=off  dbl_ovrd=off  show_param=off
      settings: xl_area=[0, 0, 0, 0, 0, 0, 0]
  Mux : xbsIndex_r3/Mux  inputs=2  precision=Full  arith_type="Signed  (2's comp)"  n_bits=8  bin_pt=2  quantization=Truncate  overflow=Wrap  latency=0  explicit_period=off  period=1  en=off  dbl_ovrd=off  show_param=off  mux_type=off  use_rpm=off  gen_core=off
      settings: xl_area=[0, 0, 0, 0, 0, 0, 0]
  Register : xbsIndex_r3/Register  init=0  reg_only_valid=off  explicit_period=off  period=1  rst=off  en=on  out_en=off  dbl_ovrd=off  show_param=off
      settings: xl_area=[0, 0, 0, 0, 0, 0, 0]
  Relational : xbsIndex_r3/Relational  mode=a>=b  latency=1  explicit_period=off  period=1  en=off  dbl_ovrd=off  show_param=off
      settings: xl_area=[0, 0, 0, 0, 0, 0, 0]
  Relational1 : xbsIndex_r3/Relational  mode=a=b  latency=1  explicit_period=on  period=1  en=off  dbl_ovrd=off  show_param=off
      settings: xl_area=[0, 0, 0, 0, 0, 0, 0]
  Slice : xbsIndex_r3/Slice  Orientation=left  mode=Lower Bit Location + Width  nbits=1  bit1=0  base1=MSB of Input  bit0=0  base0=LSB of Input  boolean_output=on  explicit_period=off  period=1  dbl_ovrd=off
  Terminator : Terminator
  pulse_extender : Subsystem  mask{pulse_len=num_elements}
      mask prompts: pulse_len "Length of Pulse"
      mask init:
      | bits = ceil(log2(pulse_len));
  pulse_extender1 : Subsystem  mask{pulse_len=num_elements}
      mask prompts: pulse_len "Length of Pulse"
      mask init:
      | bits = ceil(log2(pulse_len));
  toggle : Subsystem  mask{num_ants=num_ants, acc_len=acc_len}
      mask prompts: num_ants "Number of Antennas"; acc_len "X Engine Accumulation Length"
      mask init:
      | toggle_len = num_ants * acc_len * 2;
      | toggle_bits = floor(log2(toggle_len)) + 1;
  x_engine_valid_mask : Subsystem  mask{num_ants=num_ants}
      mask prompts: num_ants "Number of Antennas"
      mask init:
      | num_taps = floor(num_ants/2) + 1;
      | cntr_bits = floor(log2(num_taps)) + 1;
      | ant_bits = floor(log2(num_ants)) + 1;
  acc_out : Outport
  valid_out : Outport  Port=2
  sync_out : Outport  Port=3
  wires:
  toggle/1(start_end) -> x_engine_valid_mask/1(start_end)
  Delay3/1 -> Counter/3, Counter2/1, Counter1/1, Delay2/1
  Constant/1 -> Counter/2
  x_engine_valid_mask/2(valid_out_inv) -> Counter/4, Mux/1, Logical1/1
  Constant1/1 -> Relational/2
  Counter/1 -> Relational/1, Slice/1, Mux/3
  x_engine_valid_mask/1(valid_out) -> Counter2/2, Logical1/2
  Logical2/1 -> Counter/1
  Slice/1 -> Logical2/2
  valid/1 -> x_engine_valid_mask/2(valid_in)
  sync/1 -> toggle/1(sync), Delay3/1, x_engine_valid_mask/3(sync)
  Relational/1 -> Logical2/1, pulse_extender1/1(in)
  Counter2/1 -> Relational1/1, Mux/2
  Relational1/1 -> pulse_extender/1(in), Register/2
  Constant2/1 -> Relational1/2
  Logical/1 -> Counter1/2, Delay1/1
  Register/1 -> Logical3/2, Logical4/1
  Constant3/1 -> Register/1
  pulse_extender/1(out) -> Logical3/1
  pulse_extender1/1(out) -> Logical4/2
  Logical4/1 -> Logical/2
  Logical3/1 -> Logical/1
  Mux/1 -> Dual Port RAM/1
  Counter1/1 -> Dual Port RAM/4
  Delay8/1 -> Dual Port RAM/2, Dual Port RAM/5
  acc/1 -> Delay8/1
  Dual Port RAM/1 -> Terminator/1
  Dual Port RAM/2 -> acc_out/1
  Constant4/1 -> Dual Port RAM/6
  Delay1/1 -> valid_out/1
  Delay2/1 -> sync_out/1
  Logical1/1 -> Dual Port RAM/3

== system correlator_library/baseline_tap/delay ==
  In1 : Inport  Port=1  LatchInput=off
  delay_slr : delay_lib/delay_slr  DelayLen=AccLen
  Out1 : Outport
  wires:
  delay_slr/1 -> Out1/1
  In1/1 -> delay_slr/1

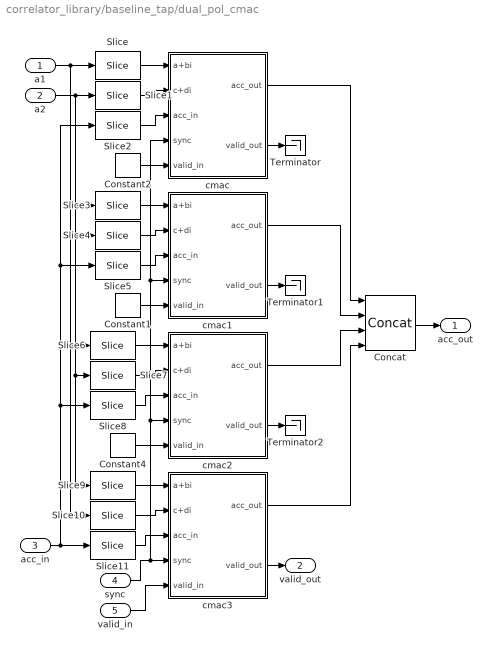
== system correlator_library/baseline_tap/dual_pol_cmac ==
  a1 : Inport  Port=1  LatchInput=off
  a2 : Inport  Port=2  LatchInput=off
  acc_in : Inport  Port=3  LatchInput=off
  sync : Inport  Port=4  LatchInput=off
  valid_in : Inport  Port=5  LatchInput=off
  Concat : xbsIndex_r3/Concat  num_inputs=4  explicit_period=off  period=1  dbl_ovrd=off
  Constant1 : xbsIndex_r3/Constant  const=0  equ=P=C  arith_type=Unsigned  n_bits=1  bin_pt=0  opselect=C  inp2=PCIN>>17  opr=+  inp1=P  carry=CIN  iostate=0  explicit_period=off  period=1  dbl_ovrd=off
  Constant2 : xbsIndex_r3/Constant  const=0  equ=P=C  arith_type=Unsigned  n_bits=1  bin_pt=0  opselect=C  inp2=PCIN>>17  opr=+  inp1=P  carry=CIN  iostate=0  explicit_period=off  period=1  dbl_ovrd=off
  Constant4 : xbsIndex_r3/Constant  const=0  equ=P=C  arith_type=Unsigned  n_bits=1  bin_pt=0  opselect=C  inp2=PCIN>>17  opr=+  inp1=P  carry=CIN  iostate=0  explicit_period=off  period=1  dbl_ovrd=off
  Slice{,1,6,9} (4 alike) : xbsIndex_r3/Slice  mode=Upper Bit Location + Width  nbits=2*BitWidthIn  bit1=0  base1=MSB of Input  bit0=0  base0=LSB of Input  boolean_output=off  explicit_period=off  period=1  dbl_ovrd=off
  Slice{3..4,7,10} (4 alike) : xbsIndex_r3/Slice  mode=Upper Bit Location + Width  nbits=2*BitWidthIn  bit1=-2*BitWidthIn  base1=MSB of Input  bit0=0  base0=LSB of Input  boolean_output=off  explicit_period=off  period=1  dbl_ovrd=off
  Slice11 : xbsIndex_r3/Slice  mode=Upper Bit Location + Width  nbits=2*BitWidthOut  bit1=-6*BitWidthOut  base1=MSB of Input  bit0=0  base0=LSB of Input  boolean_output=off  explicit_period=off  period=1  dbl_ovrd=off
  Slice2 : xbsIndex_r3/Slice  mode=Upper Bit Location + Width  nbits=2*BitWidthOut  bit1=0  base1=MSB of Input  bit0=0  base0=LSB of Input  boolean_output=off  explicit_period=off  period=1  dbl_ovrd=off
  Slice5 : xbsIndex_r3/Slice  mode=Upper Bit Location + Width  nbits=2*BitWidthOut  bit1=-2*BitWidthOut  base1=MSB of Input  bit0=0  base0=LSB of Input  boolean_output=off  explicit_period=off  period=1  dbl_ovrd=off
  Slice8 : xbsIndex_r3/Slice  mode=Upper Bit Location + Width  nbits=2*BitWidthOut  bit1=-4*BitWidthOut  base1=MSB of Input  bit0=0  base0=LSB of Input  boolean_output=off  explicit_period=off  period=1  dbl_ovrd=off
  Terminator : Terminator
  Terminator1 : Terminator
  Terminator2 : Terminator
  cmac : Subsystem
  cmac1 : Subsystem
  cmac2 : Subsystem
  cmac3 : Subsystem
  acc_out : Outport
  valid_out : Outport  Port=2
  wires:
  Slice/1 -> cmac/1(a+bi)
  Slice1/1 -> cmac/2(c+di)
  Slice2/1 -> cmac/3(acc_in)
  Slice3/1 -> cmac1/1(a+bi)
  Slice4/1 -> cmac1/2(c+di)
  Slice5/1 -> cmac1/3(acc_in)
  Concat/1 -> acc_out/1
  Constant2/1 -> cmac/5(valid_in)
  cmac/2(valid_out) -> Terminator/1
  Constant1/1 -> cmac1/5(valid_in)
  Slice6/1 -> cmac2/1(a+bi)
  Slice7/1 -> cmac2/2(c+di)
  Slice8/1 -> cmac2/3(acc_in)
  Constant4/1 -> cmac2/5(valid_in)
  Slice9/1 -> cmac3/1(a+bi)
  Slice10/1 -> cmac3/2(c+di)
  Slice11/1 -> cmac3/3(acc_in)
  valid_in/1 -> cmac3/5(valid_in)
  sync/1 -> cmac/4(sync), cmac1/4(sync), cmac2/4(sync), cmac3/4(sync)
  cmac1/2(valid_out) -> Terminator1/1
  cmac2/2(valid_out) -> Terminator2/1
  cmac3/2(valid_out) -> valid_out/1
  cmac/1(acc_out) -> Concat/1
  cmac1/1(acc_out) -> Concat/2
  cmac2/1(acc_out) -> Concat/3
  cmac3/1(acc_out) -> Concat/4
  a1/1 -> Slice/1, Slice3/1, Slice6/1, Slice10/1
  a2/1 -> Slice1/1, Slice4/1, Slice7/1, Slice9/1
  acc_in/1 -> Slice11/1, Slice8/1, Slice5/1, Slice2/1

== system correlator_library/vacc/acc_core ==
  din : Inport  Port=1  LatchInput=off
  we : Inport  Port=2  LatchInput=off
  rst : Inport  Port=3  LatchInput=off
  re : Inport  Port=4  LatchInput=off
  acc_en : Inport  Port=5  LatchInput=off
  const0 : xbsIndex_r3/Constant  const=0  equ=P=C  arith_type=Unsigned  n_bits=n_bits  bin_pt=bin_pt  opselect=C  inp2=PCIN>>17  opr=+  inp1=P  carry=CIN  iostate=0  explicit_period=on  period=1  dbl_ovrd=off
  const1 : xbsIndex_r3/Constant  const=0  equ=P=C  arith_type=Boolean  n_bits=1  bin_pt=0  opselect=C  inp2=PCIN>>17  opr=+  inp1=P  carry=CIN  iostate=0  explicit_period=on  period=1  dbl_ovrd=off
  vacc_fifo1 : correlator_library/vacc_fifo  vlen=vlen  n_bits=n_bits  bin_pt=bin_pt  add_latency=add_latency  arith_type=Unsigned  BitWidthIn=BitWidthIn  BinPtIn=BinPtIn  streams=streams  stream=1
      link override constant: equ=P=C  arith_type=Unsigned
  vacc_fifo2 : correlator_library/vacc_fifo  vlen=vlen  n_bits=n_bits  bin_pt=bin_pt  add_latency=add_latency  arith_type=Unsigned  BitWidthIn=BitWidthIn  BinPtIn=BinPtIn  streams=streams  stream=2
      link override constant: equ=P=C
  dout : Outport
  valid : Outport  Port=2
  empty : Outport  Port=3
  wires:
  vacc_fifo2/8 -> empty/1
  vacc_fifo2/4 -> valid/1
  vacc_fifo2/3 -> dout/1
  acc_en/1 -> vacc_fifo1/7
  re/1 -> vacc_fifo1/6
  rst/1 -> vacc_fifo1/5
  const1/1 -> vacc_fifo1/4
  const0/1 -> vacc_fifo1/3
  we/1 -> vacc_fifo1/2
  din/1 -> vacc_fifo1/1
  vacc_fifo1/7 -> vacc_fifo2/7
  vacc_fifo1/6 -> vacc_fifo2/6
  vacc_fifo1/5 -> vacc_fifo2/5
  vacc_fifo1/4 -> vacc_fifo2/4
  vacc_fifo1/3 -> vacc_fifo2/3
  vacc_fifo1/2 -> vacc_fifo2/2
  vacc_fifo1/1 -> vacc_fifo2/1

== system correlator_library/vacc/freeze_cntr1 ==
  rst : Inport  Port=1  LatchInput=off
  Constant5 : xbsIndex_r3/Constant  const=2^CounterBits - 2  equ=P=C  arith_type=Unsigned  n_bits=CounterBits  bin_pt=0  opselect=C  inp2=PCIN>>17  opr=+  inp1=P  carry=CIN  iostate=0  explicit_period=off  period=1  dbl_ovrd=off
  Counter3 : xbsIndex_r3/Counter  cnt_type=Free Running  n_bits=CounterBits  bin_pt=0  arith_type=Unsigned  start_count=0  cnt_to=1023  cnt_by_val=1  operation=Up  explicit_period=on  period=1  load_pin=off  rst=on  en=on  dbl_ovrd=off  show_param=off  use_rpm=on  gen_core=off
      settings: xl_area=[0, 0, 0, 0, 0, 0, 0]
  Delay : xbsIndex_r3/Delay  latency=1  reg_retiming=off  explicit_period=off  period=1  en=off  accept_only_valid=off  init_zero=on  dbl_ovrd=off  show_param=off
      settings: xl_area=[0, 0, 0, 0, 0, 0, 0]
  Inverter : xbsIndex_r3/Inverter  latency=0  explicit_period=off  period=1  en=off  dbl_ovrd=off  show_param=off
      settings: xl_area=[0, 0, 0, 0, 0, 0, 0]
  Logical1 : xbsIndex_r3/Logical  logical_function=AND  inputs=2  precision=Full  arith_type=Unsigned  n_bits=8  bin_pt=2  align_bp=on  latency=0  explicit_period=off  period=1  en=off  dbl_ovrd=off  show_param=off
      settings: xl_area=[0, 0, 0, 0, 0, 0, 0]
  Logical2 : xbsIndex_r3/Logical  logical_function=OR  inputs=2  precision=Full  arith_type=Unsigned  n_bits=8  bin_pt=2  align_bp=on  latency=0  explicit_period=off  period=1  en=off  dbl_ovrd=off  show_param=off
      settings: xl_area=[0, 0, 0, 0, 0, 0, 0]
  Logical3 : xbsIndex_r3/Logical  logical_function=OR  inputs=2  precision=Full  arith_type=Unsigned  n_bits=8  bin_pt=2  align_bp=on  latency=0  explicit_period=off  period=1  en=off  dbl_ovrd=off  show_param=off
      settings: xl_area=[0, 0, 0, 0, 0, 0, 0]
  Relational5 : xbsIndex_r3/Relational  mode=a<b  latency=1  explicit_period=off  period=1  en=off  dbl_ovrd=off  show_param=off
      settings: xl_area=[0, 0, 0, 0, 0, 0, 0]
  negedge : Subsystem
  addr : Outport
  we : Outport  Port=2
  wires:
  Counter3/1 -> addr/1, Relational5/1
  Constant5/1 -> Relational5/2
  rst/1 -> Counter3/1, Inverter/1, negedge/1(in)
  Logical1/1 -> we/1
  Inverter/1 -> Logical1/1
  Logical3/1 -> Counter3/2, Logical2/2, Delay/1
  Relational5/1 -> Logical3/2
  negedge/1(out) -> Logical3/1
  Logical2/1 -> Logical1/2
  Delay/1 -> Logical2/1

== system correlator_library/vacc/posedge ==
  in : Inport  Port=1  LatchInput=off
  Delay : xbsIndex_r3/Delay  latency=1  reg_retiming=off  explicit_period=off  period=1  en=off  accept_only_valid=off  init_zero=on  dbl_ovrd=off  show_param=off
      settings: xl_area=[0, 0, 0, 0, 0, 0, 0]
  Inverter : xbsIndex_r3/Inverter  latency=0  explicit_period=off  period=1  en=off  dbl_ovrd=off  show_param=off
      settings: xl_area=[0, 0, 0, 0, 0, 0, 0]
  Logical : xbsIndex_r3/Logical  logical_function=AND  inputs=2  precision=Full  arith_type=Unsigned  n_bits=8  bin_pt=2  align_bp=on  latency=0  explicit_period=off  period=1  en=off  dbl_ovrd=off  show_param=off
      settings: xl_area=[0, 0, 0, 0, 0, 0, 0]
  out : Outport
  wires:
  Delay/1 -> Inverter/1
  Inverter/1 -> Logical/1
  in/1 -> Delay/1, Logical/2
  Logical/1 -> out/1

== system correlator_library/vacc_fifo/posedge ==
  in : Inport  Port=1  LatchInput=off
  Delay : xbsIndex_r3/Delay  latency=1  reg_retiming=off  explicit_period=off  period=1  en=off  accept_only_valid=off  init_zero=on  dbl_ovrd=off  show_param=off
      settings: xl_area=[0, 0, 0, 0, 0, 0, 0]
  Inverter : xbsIndex_r3/Inverter  latency=0  explicit_period=off  period=1  en=off  dbl_ovrd=off  show_param=off
      settings: xl_area=[0, 0, 0, 0, 0, 0, 0]
  Logical : xbsIndex_r3/Logical  logical_function=AND  inputs=2  precision=Full  arith_type=Unsigned  n_bits=8  bin_pt=2  align_bp=on  latency=0  explicit_period=off  period=1  en=off  dbl_ovrd=off  show_param=off
      settings: xl_area=[0, 0, 0, 0, 0, 0, 0]
  out : Outport
  wires:
  Delay/1 -> Inverter/1
  Inverter/1 -> Logical/1
  in/1 -> Delay/1, Logical/2
  Logical/1 -> out/1
